simulink model "DMC_plant_velocity"  (R2022b)
settings: Solver=ode4  StartTime=0.0  StopTime=100  FixedStep=0.1  RelTol=1e-3  EnableMultiTasking=on
Description:
  | Real-Time Van der Pol Simulation
  | 
  | This demonstration shows a real-time version of the Simulink Van der Pol
  | simulation demo. This model does not need any external signals, so it does
  | not need any data acquisition hardware or driver. This makes the model ideal
  | for first experiments with Real-Time Windows Target, without need to
  | worry about proper I/O hardware configuration.
  | 
  | How to run this demo:
  | 
  |   1. Build the model using Tools -> Real-Time Workshop -> Build Model.
  |   2. Connect to the real-time code using Simulation -> Connect to target.
  |   3. Start the real-time execution using Simulation -> Start real-time code.
settings Model: SimulationMode=external  Creator=Houska  LastModifiedBy=artur
settings SolverCC: AlgebraicLoopSolver=TrustRegion
settings DataIOCC: LimitDataPoints=on  SaveFormat=Array  SignalLoggingSaveFormat=ModelDataLogs  SaveOutput=off  SaveTime=off  ReturnWorkspaceOutputs=off  SignalLoggingName=logsOut
settings OptimizationCC: ExpressionDepthLimit=2147483647  InitFltsAndDblsToZero=on
settings DebuggingCC: SaveWithParameterizedLinksMsg=none  UnderspecifiedInitializationDetection=Classic  MergeDetectMultiDrivingBlocksExec=none  SignalResolutionControl=TryResolveAllWithWarning  MultiTaskDSMMsg=warning  MultiTaskCondExecSysMsg=none  FcnCallInpInsideContextMsg=warning  UnconnectedInputMsg=warning  UnconnectedOutputMsg=warning  UnconnectedLineMsg=warning  AllowSymbolicDim=off  StateNameClashWarn=warning  PregeneratedLibrarySubsystemCodeDiagnostic=none  SFUnexpectedBacktrackingDiag=warning  SFNoUnconditionalDefaultTransitionDiag=warning  SFExecutionAtInitializationDiag=none  SFMachineParentedDataDiag=warning  ArithmeticOperatorsInVariantConditions=warning
settings HardwareCC: ProdBitPerPointer=32  ProdBitPerSizeT=32  ProdBitPerPtrDiffT=32  ProdLargestAtomicFloat=None  ProdWordSize=32  ProdHWDeviceType=32-bit Real-Time Windows Target  TargetHWDeviceType=32-bit Generic  ProdEqTarget=off
settings ModelReferenceCC: EnableRefExpFcnMdlSchedulingChecks=on  PropagateSignalLabelsOutOfModel=off
settings SFSimCC: SimUseLocalCustomCode=off  CustomCodeUndefinedFunction=UseInterfaceOnly
settings RTWCC: Description=servo (Visual C/C++)  SystemTargetFile=rtcon_servo_usb2.tlc  TemplateMakefile=servo_vc_usb2_x64.tmf  RTWUseLocalCustomCode=off  DLArmComputeVersion=19.05
settings CodeAppCC: StateflowObjectComments=on
settings STFCustomTargetCC: ModelReferenceCompliant=off  CombineOutputUpdateFcns=on  MatFileLogging=on  SystemTargetFile=rtcon_servo_usb2.tlc
settings GRTTargetCC: TargetLangStandard=C89/C90 (ANSI)  ModelReferenceCompliant=off  ParMdlRefBuildCompliant=off  CompOptLevelCompliant=off  ConcurrentExecutionCompliant=off  CPPClassGenCompliant=off  UseToolchainInfoCompliant=off  ExtMode=on  ExtModeMexFile=rtcon_ext_comm
settings ConfigComp: CovMetricSettings=dw  CovSaveCumulativeToWorkspaceVar=on  CovSaveSingleToWorkspaceVar=on  CovExternalEMLEnable=off  CovSFcnEnable=off

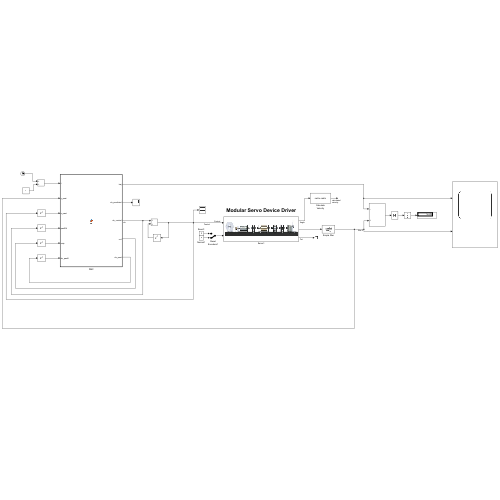
[thumbnail: Simulink's stored preview of the top-level diagram]
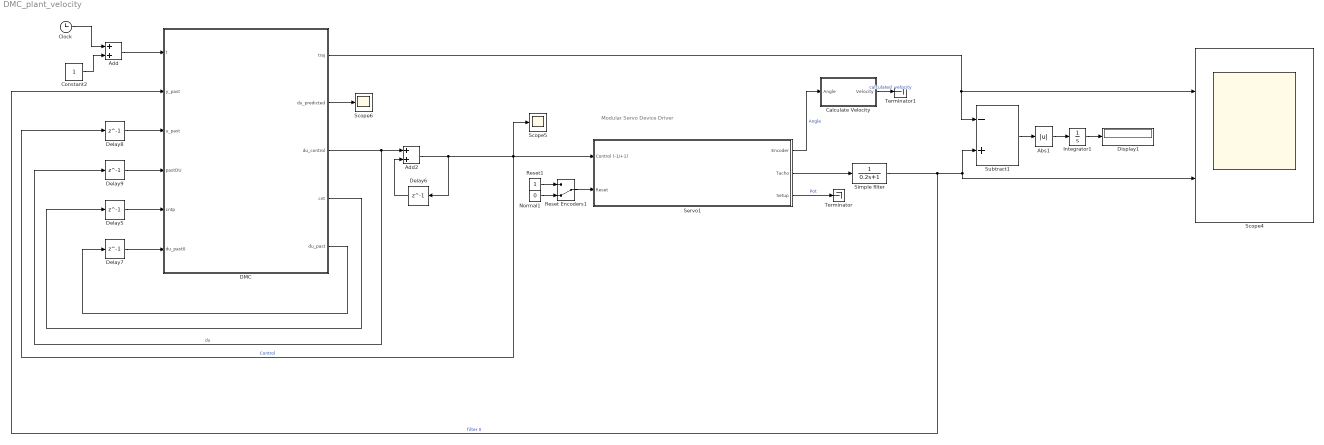
== system DMC_plant_velocity ==
  note: Modular Servo Device Driver
  Abs1 : Abs  SaturateOnIntegerOverflow=off
  Add : Sum
  Add2 : Sum
  Calculate Velocity : Subsystem
      mask Display: disp( 'rad-to-rad/s' )
  Clock : Clock
  Constant2 : Constant
  DMC : MATLAB Function  TreatAsAtomicUnit=on
  Delay5 : Delay  DelayLength=1  InitialCondition=1
  Delay6 : Delay  DelayLength=1  InitialCondition=0
  Delay7 : Delay  DelayLength=1  InitialCondition=zeros(1,150-1)
  Delay8 : Delay  DelayLength=1  InitialCondition=0
  Delay9 : Delay  DelayLength=1  InitialCondition=0
  Display1 : Display
  Integrator1 : Integrator
  Normal1 : Constant  Value=0
  Reset Encoders1 : ManualSwitch  CurrentSetting=0
  Reset1 : Constant
  Scope4 : Scope  NumInputPorts=2
  Scope5 : Scope
  Scope6 : Scope
  Servo1 : Subsystem
      mask Display: image(imread('Servo_inteco.JPG'))
  Simple filter : TransferFcn  Denominator=[0.2 1]
  Subtract1 : Sum  Inputs=-+
  Terminator : Terminator
  Terminator1 : Terminator
  wires:
  Delay8/1 -> DMC/3(u_past)
  Add/1 -> DMC/1(t)
  Integrator1/1 -> Display1/1
  Delay7/1 -> DMC/6(du_past0)
  Delay5/1 -> DMC/5(cntp)
  DMC/2(du_predicted) -> Scope6/1
  DMC/5(du_past) -> Delay7/1
  Servo1/2(Tacho) -> Simple filter/1
  DMC/3(du_control) -> Add2/1, Delay9/1  "du"
  Servo1/1(Encoder) -> Calculate Velocity/1(Angle)  "Angle"
  DMC/4(cnt) -> Delay5/1
  Delay6/1 -> Add2/2
  Delay9/1 -> DMC/4(pastDU)
  Abs1/1 -> Integrator1/1
  Subtract1/1 -> Abs1/1
  DMC/1(traj) -> Scope4/1, Subtract1/1
  Add2/1 -> Delay6/1, Servo1/1(Control (-1/+1)), Scope5/1, Delay8/1  "Control"
  Normal1/1 -> Reset Encoders1/2
  Reset1/1 -> Reset Encoders1/1
  Reset Encoders1/1 -> Servo1/2(Reset)
  Servo1/3(Setup) -> Terminator/1  "Pot"
  Constant2/1 -> Add/2
  Clock/1 -> Add/1
  Calculate Velocity/1(Velocity) -> Terminator1/1  "calculated  velocity"
  Simple filter/1 -> DMC/2(y_past), Scope4/2, Subtract1/2  "filter II"

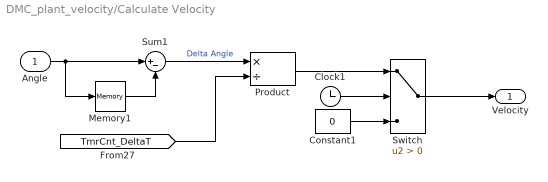
== system DMC_plant_velocity/Calculate Velocity ==
  Angle : Inport
  Clock1 : Clock
  Constant1 : Constant  Value=0
  Memory1 : Memory
  Product : Product  Inputs=*/  InputSameDT=on  SaturateOnIntegerOverflow=on  OutDataTypeStr=Inherit: Same as first input
  Sum1 : Sum  Inputs=|+-  InputSameDT=on  SaturateOnIntegerOverflow=on  OutDataTypeStr=Inherit: Same as first input
  Switch : Switch  Criteria=u2 > Threshold
  Velocity : Outport  VectorParamsAs1DForOutWhenUnconnected=off
  wires:
  Switch/1 -> Velocity/1
  Constant1/1 -> Switch/3
  Clock1/1 -> Switch/2
  Product/1 -> Switch/1
  Sum1/1 -> Product/1  "Delta Angle"
  Angle/1 -> Memory1/1, Sum1/1
  Memory1/1 -> Sum1/2
  [TmrCnt_DeltaT] -> Product/2

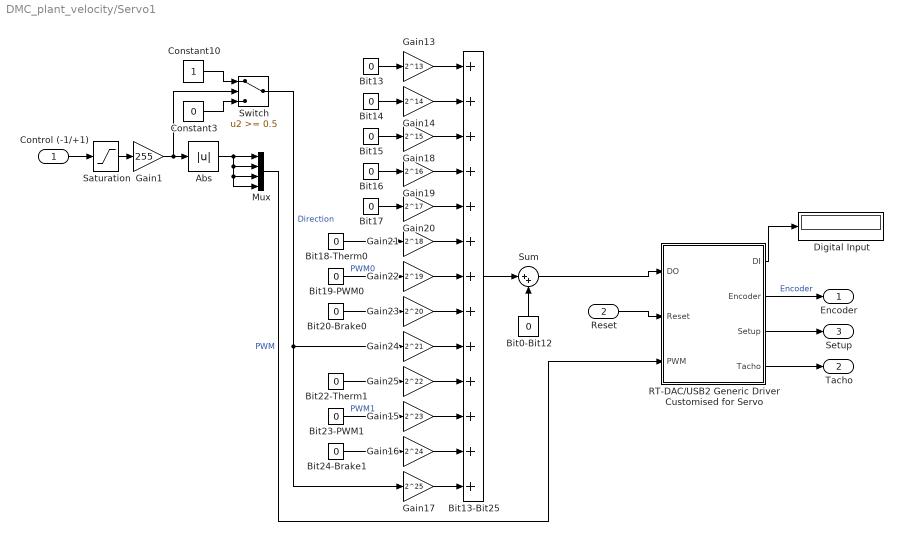
== system DMC_plant_velocity/Servo1 ==
  Control (-1/+1) : Inport
  Reset : Inport  Port=2
  Abs : Abs
  Bit0-Bit12 : Constant  Value=0
  Bit{13..17} (5 alike) : Constant  Value=0
  Bit13-Bit25 : Sum  Inputs=+++++++++++++  InputSameDT=on  SaturateOnIntegerOverflow=on  OutDataTypeStr=Inherit: Same as first input
  Bit18-Therm0 : Constant  Value=0
  Bit19-PWM0 : Constant  Value=0
  Bit20-Brake0 : Constant  Value=0
  Bit22-Therm1 : Constant  Value=0
  Bit23-PWM1 : Constant  Value=0
  Bit24-Brake1 : Constant  Value=0
  Constant10 : Constant
  Constant3 : Constant  Value=0
  Digital Input : Display
  Gain1 : Gain  Gain=255  SaturateOnIntegerOverflow=on  OutDataTypeStr=Inherit: Same as input  ParamDataTypeStr=Inherit: Same as input
  Gain13 : Gain  Gain=2^13  SaturateOnIntegerOverflow=on  OutDataTypeStr=Inherit: Same as input  ParamDataTypeStr=Inherit: Same as input
  Gain14 : Gain  Gain=2^14  SaturateOnIntegerOverflow=on  OutDataTypeStr=Inherit: Same as input  ParamDataTypeStr=Inherit: Same as input
  Gain15 : Gain  Gain=2^23  SaturateOnIntegerOverflow=on  OutDataTypeStr=Inherit: Same as input  ParamDataTypeStr=Inherit: Same as input
  Gain16 : Gain  Gain=2^24  SaturateOnIntegerOverflow=on  OutDataTypeStr=Inherit: Same as input  ParamDataTypeStr=Inherit: Same as input
  Gain17 : Gain  Gain=2^25  SaturateOnIntegerOverflow=on  OutDataTypeStr=Inherit: Same as input  ParamDataTypeStr=Inherit: Same as input
  Gain18 : Gain  Gain=2^15  SaturateOnIntegerOverflow=on  OutDataTypeStr=Inherit: Same as input  ParamDataTypeStr=Inherit: Same as input
  Gain19 : Gain  Gain=2^16  SaturateOnIntegerOverflow=on  OutDataTypeStr=Inherit: Same as input  ParamDataTypeStr=Inherit: Same as input
  Gain20 : Gain  Gain=2^17  SaturateOnIntegerOverflow=on  OutDataTypeStr=Inherit: Same as input  ParamDataTypeStr=Inherit: Same as input
  Gain21 : Gain  Gain=2^18  SaturateOnIntegerOverflow=on  OutDataTypeStr=Inherit: Same as input  ParamDataTypeStr=Inherit: Same as input
  Gain22 : Gain  Gain=2^19  SaturateOnIntegerOverflow=on  OutDataTypeStr=Inherit: Same as input  ParamDataTypeStr=Inherit: Same as input
  Gain23 : Gain  Gain=2^20  SaturateOnIntegerOverflow=on  OutDataTypeStr=Inherit: Same as input  ParamDataTypeStr=Inherit: Same as input
  Gain24 : Gain  Gain=2^21  SaturateOnIntegerOverflow=on  OutDataTypeStr=Inherit: Same as input  ParamDataTypeStr=Inherit: Same as input
  Gain25 : Gain  Gain=2^22  SaturateOnIntegerOverflow=on  OutDataTypeStr=Inherit: Same as input  ParamDataTypeStr=Inherit: Same as input
  Mux : Mux
  RT-DAC/USB2 Generic Driver Customised for Servo : Subsystem
      mask Display: disp('RT-DAC/USB2\n\nGeneric Driver\nVersion 2.1')
  Saturation : Saturate  UpperLimit=1  LowerLimit=-1
  Sum : Sum  Inputs=|++  InputSameDT=on  SaturateOnIntegerOverflow=on  OutDataTypeStr=Inherit: Same as first input
  Switch : Switch  Threshold=0.5  SaturateOnIntegerOverflow=off
  Encoder : Outport  VectorParamsAs1DForOutWhenUnconnected=off
  Tacho : Outport  Port=2  VectorParamsAs1DForOutWhenUnconnected=off
  Setup : Outport  Port=3  VectorParamsAs1DForOutWhenUnconnected=off
  wires:
  RT-DAC/USB2 Generic Driver Customised for Servo/4(Tacho) -> Tacho/1
  RT-DAC/USB2 Generic Driver Customised for Servo/3(Setup) -> Setup/1
  RT-DAC/USB2 Generic Driver Customised for Servo/2(Encoder) -> Encoder/1  "Encoder"
  Mux/1 -> RT-DAC/USB2 Generic Driver Customised for Servo/3(PWM)  "PWM"
  Switch/1 -> Gain17/1, Gain24/1  "Direction"
  Abs/1 -> Mux/4, Mux/3, Mux/2, Mux/1
  Constant3/1 -> Switch/3
  Constant10/1 -> Switch/1
  Gain1/1 -> Switch/2, Abs/1
  Saturation/1 -> Gain1/1
  Control (-1/+1)/1 -> Saturation/1
  Reset/1 -> RT-DAC/USB2 Generic Driver Customised for Servo/2(Reset)
  Bit24-Brake1/1 -> Gain16/1
  Bit23-PWM1/1 -> Gain15/1  "PWM1"
  Bit22-Therm1/1 -> Gain25/1
  Bit13-Bit25/1 -> Sum/1
  Sum/1 -> RT-DAC/USB2 Generic Driver Customised for Servo/1(DO)
  Gain17/1 -> Bit13-Bit25/13
  Gain16/1 -> Bit13-Bit25/12
  Gain15/1 -> Bit13-Bit25/11
  Gain25/1 -> Bit13-Bit25/10
  Gain24/1 -> Bit13-Bit25/9
  Gain23/1 -> Bit13-Bit25/8
  Gain22/1 -> Bit13-Bit25/7
  Gain21/1 -> Bit13-Bit25/6
  Gain20/1 -> Bit13-Bit25/5
  Gain19/1 -> Bit13-Bit25/4
  Gain18/1 -> Bit13-Bit25/3
  Gain14/1 -> Bit13-Bit25/2
  Gain13/1 -> Bit13-Bit25/1
  Bit0-Bit12/1 -> Sum/2
  RT-DAC/USB2 Generic Driver Customised for Servo/1(DI) -> Digital Input/1
  Bit20-Brake0/1 -> Gain23/1
  Bit19-PWM0/1 -> Gain22/1  "PWM0"
  Bit18-Therm0/1 -> Gain21/1
  Bit17/1 -> Gain20/1
  Bit16/1 -> Gain19/1
  Bit15/1 -> Gain18/1
  Bit14/1 -> Gain14/1
  Bit13/1 -> Gain13/1

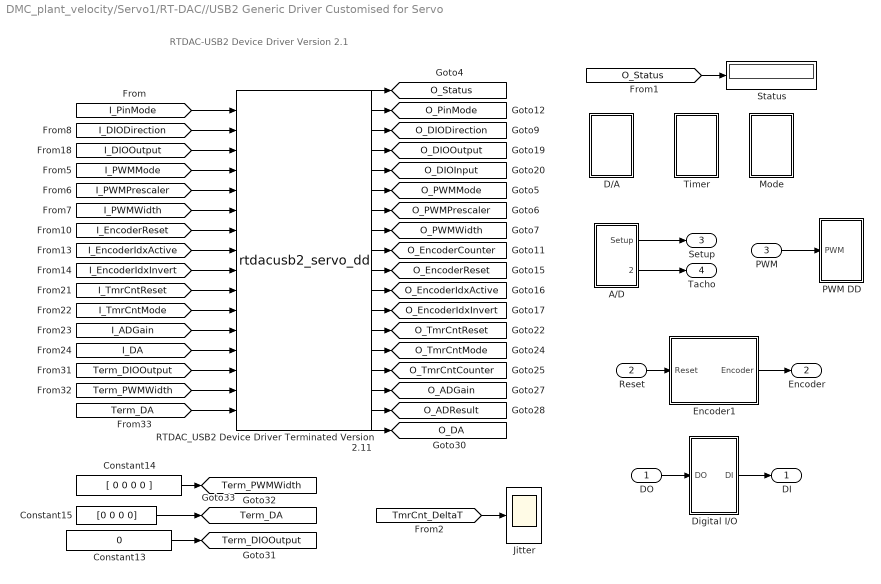
== system DMC_plant_velocity/Servo1/RT-DAC//USB2 Generic Driver Customised for Servo ==
  note: RTDAC-USB2 Device Driver
      | Version 2.1
  DO : Inport
  Reset : Inport  Port=2
  PWM : Inport  Port=3
  A/D : Subsystem
  Constant13 : Constant  Value=0
  Constant14 : Constant  Value=[ 0 0 0 0 ]
  Constant15 : Constant  Value=[0 0 0 0]
  D/A : Subsystem
  Digital I/O : Subsystem
  Encoder1 : Subsystem
  Jitter : Scope
  Mode : Subsystem
  PWM DD : Subsystem
  RTDAC_USB2 Device Driver Terminated Version 2.11 : S-Function  FunctionName=rtdacusb2_servo_dd  Parameters=0.1  SFunctionDeploymentMode=off  EnableBusSupport=off
  Status : Display
  Timer : Subsystem
  DI : Outport  VectorParamsAs1DForOutWhenUnconnected=off
  Encoder : Outport  Port=2  VectorParamsAs1DForOutWhenUnconnected=off
  Setup : Outport  Port=3  VectorParamsAs1DForOutWhenUnconnected=off
  Tacho : Outport  Port=4  VectorParamsAs1DForOutWhenUnconnected=off
  tag scope: O_ADGain=global, O_ADResult=global, O_DA=global, O_DIODirection=global, O_DIOInput=global, O_DIOOutput=global, O_EncoderCounter=global, O_EncoderIdxActive=global, O_EncoderIdxInvert=global, O_EncoderReset=global, O_PWMMode=global, O_PWMPrescaler=global, O_PWMWidth=global, O_PinMode=global, O_Status=global, O_TmrCntCounter=global, O_TmrCntMode=global, O_TmrCntReset=global, Term_DA=global, Term_DIOOutput=global, Term_PWMWidth=global
  wires:
  [TmrCnt_DeltaT] -> Jitter/1
  Constant14/1 -> [Term_PWMWidth]
  [Term_DA] -> RTDAC_USB2 Device Driver Terminated Version 2.11/16
  [Term_PWMWidth] -> RTDAC_USB2 Device Driver Terminated Version 2.11/15
  [Term_DIOOutput] -> RTDAC_USB2 Device Driver Terminated Version 2.11/14
  Constant13/1 -> [Term_DIOOutput]
  Constant15/1 -> [Term_DA]
  A/D/2(Tacho) -> Tacho/1
  A/D/1(Setup) -> Setup/1
  Reset/1 -> Encoder1/1(Reset)
  Digital I/O/1(DI) -> DI/1
  DO/1 -> Digital I/O/1(DO)
  Encoder1/1(Encoder) -> Encoder/1
  RTDAC_USB2 Device Driver Terminated Version 2.11/5 -> [O_DIOInput]
  RTDAC_USB2 Device Driver Terminated Version 2.11/4 -> [O_DIOOutput]
  [I_DIOOutput] -> RTDAC_USB2 Device Driver Terminated Version 2.11/3
  RTDAC_USB2 Device Driver Terminated Version 2.11/12 -> [O_EncoderIdxInvert]
  RTDAC_USB2 Device Driver Terminated Version 2.11/11 -> [O_EncoderIdxActive]
  RTDAC_USB2 Device Driver Terminated Version 2.11/10 -> [O_EncoderReset]
  [I_EncoderIdxInvert] -> RTDAC_USB2 Device Driver Terminated Version 2.11/9
  [I_EncoderIdxActive] -> RTDAC_USB2 Device Driver Terminated Version 2.11/8
  RTDAC_USB2 Device Driver Terminated Version 2.11/2 -> [O_PinMode]
  RTDAC_USB2 Device Driver Terminated Version 2.11/3 -> [O_DIODirection]
  RTDAC_USB2 Device Driver Terminated Version 2.11/9 -> [O_EncoderCounter]
  [I_EncoderReset] -> RTDAC_USB2 Device Driver Terminated Version 2.11/7
  [I_DIODirection] -> RTDAC_USB2 Device Driver Terminated Version 2.11/2
  [I_PWMWidth] -> RTDAC_USB2 Device Driver Terminated Version 2.11/6
  [I_PWMPrescaler] -> RTDAC_USB2 Device Driver Terminated Version 2.11/5
  [I_PWMMode] -> RTDAC_USB2 Device Driver Terminated Version 2.11/4
  RTDAC_USB2 Device Driver Terminated Version 2.11/8 -> [O_PWMWidth]
  RTDAC_USB2 Device Driver Terminated Version 2.11/7 -> [O_PWMPrescaler]
  RTDAC_USB2 Device Driver Terminated Version 2.11/6 -> [O_PWMMode]
  [O_Status] -> Status/1
  RTDAC_USB2 Device Driver Terminated Version 2.11/1 -> [O_Status]
  PWM/1 -> PWM DD/1(PWM)
  [I_PinMode] -> RTDAC_USB2 Device Driver Terminated Version 2.11/1
  [I_TmrCntReset] -> RTDAC_USB2 Device Driver Terminated Version 2.11/10
  [I_ADGain] -> RTDAC_USB2 Device Driver Terminated Version 2.11/12
  [I_TmrCntMode] -> RTDAC_USB2 Device Driver Terminated Version 2.11/11
  [I_DA] -> RTDAC_USB2 Device Driver Terminated Version 2.11/13
  RTDAC_USB2 Device Driver Terminated Version 2.11/13 -> [O_TmrCntReset]
  RTDAC_USB2 Device Driver Terminated Version 2.11/14 -> [O_TmrCntMode]
  RTDAC_USB2 Device Driver Terminated Version 2.11/15 -> [O_TmrCntCounter]
  RTDAC_USB2 Device Driver Terminated Version 2.11/16 -> [O_ADGain]
  RTDAC_USB2 Device Driver Terminated Version 2.11/17 -> [O_ADResult]
  RTDAC_USB2 Device Driver Terminated Version 2.11/18 -> [O_DA]

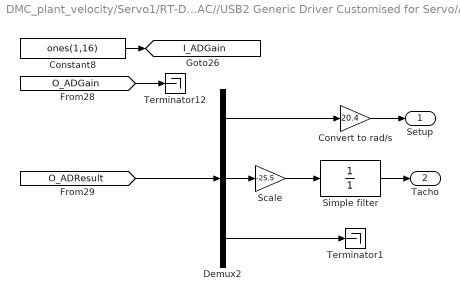
== system DMC_plant_velocity/Servo1/RT-DAC//USB2 Generic Driver Customised for Servo/A//D ==
  Constant8 : Constant  Value=ones(1,16)
  Convert to rad/s : Gain  Gain=20.4  OutDataTypeStr=Inherit: Same as input  ParamDataTypeStr=Inherit: Same as input
  Demux2 : Demux  Outputs=[1 1 14]
      settings: DisplayOption=none
  Scale : Gain  Gain=-25.5  OutDataTypeStr=Inherit: Same as input  ParamDataTypeStr=Inherit: Same as input
  Simple filter : TransferFcn  Denominator=[0.0 1]
  Terminator1 : Terminator
  Terminator12 : Terminator
  Setup : Outport  InitialOutput=0  VectorParamsAs1DForOutWhenUnconnected=off
  Tacho : Outport  Port=2  InitialOutput=0  VectorParamsAs1DForOutWhenUnconnected=off
  tag scope: I_ADGain=global
  wires:
  Scale/1 -> Simple filter/1
  Demux2/3 -> Terminator1/1
  Simple filter/1 -> Tacho/1
  Convert to rad/s/1 -> Setup/1
  Demux2/1 -> Convert to rad/s/1
  Demux2/2 -> Scale/1
  Constant8/1 -> [I_ADGain]
  [O_ADGain] -> Terminator12/1
  [O_ADResult] -> Demux2/1

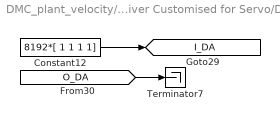
== system DMC_plant_velocity/Servo1/RT-DAC//USB2 Generic Driver Customised for Servo/D//A ==
  Constant12 : Constant  Value=8192*[ 1 1 1 1]
  Terminator7 : Terminator
  tag scope: I_DA=global
  wires:
  [O_DA] -> Terminator7/1
  Constant12/1 -> [I_DA]

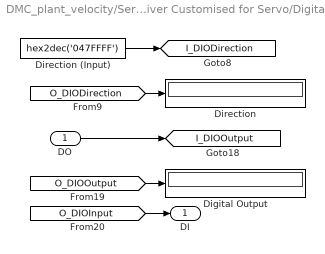
== system DMC_plant_velocity/Servo1/RT-DAC//USB2 Generic Driver Customised for Servo/Digital I//O ==
  DO : Inport
  Digital Output : Display
  Direction : Display
  Direction (Input) : Constant  Value=hex2dec('047FFFF')
  DI : Outport  VectorParamsAs1DForOutWhenUnconnected=off
  tag scope: I_DIODirection=global, I_DIOOutput=global
  wires:
  [O_DIOInput] -> DI/1
  [O_DIOOutput] -> Digital Output/1
  DO/1 -> [I_DIOOutput]
  [O_DIODirection] -> Direction/1
  Direction (Input)/1 -> [I_DIODirection]

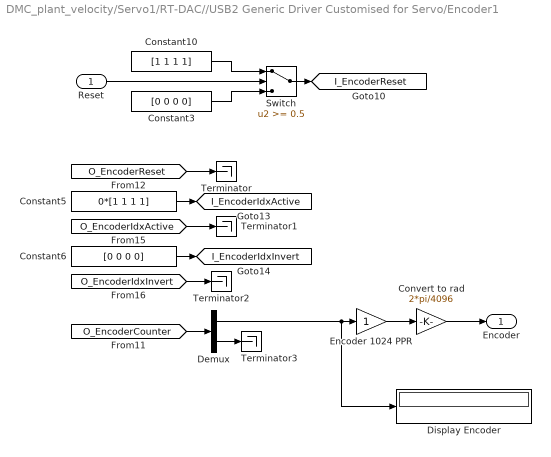
== system DMC_plant_velocity/Servo1/RT-DAC//USB2 Generic Driver Customised for Servo/Encoder1 ==
  Reset : Inport
  Constant10 : Constant  Value=[1 1 1 1]
  Constant3 : Constant  Value=[0 0 0 0]
  Constant5 : Constant  Value=0*[1 1 1 1]
  Constant6 : Constant  Value=[0 0 0 0]
  Convert to rad : Gain  Gain=2*pi/4096  SaturateOnIntegerOverflow=on  OutDataTypeStr=Inherit: Same as input  ParamDataTypeStr=Inherit: Same as input
  Demux : Demux  Outputs=[1 3]
  Display Encoder : Display
  Encoder 1024 PPR : Gain  SaturateOnIntegerOverflow=on  OutDataTypeStr=Inherit: Same as input  ParamDataTypeStr=Inherit: Same as input
  Switch : Switch  Threshold=0.5  SaturateOnIntegerOverflow=off
  Terminator{,1..3} (4 alike) : Terminator
  Encoder : Outport  VectorParamsAs1DForOutWhenUnconnected=off
  tag scope: I_EncoderIdxActive=global, I_EncoderIdxInvert=global, I_EncoderReset=global
  wires:
  Convert to rad/1 -> Encoder/1
  Demux/1 -> Encoder 1024 PPR/1, Display Encoder/1
  Encoder 1024 PPR/1 -> Convert to rad/1
  Reset/1 -> Switch/2
  Constant3/1 -> Switch/3
  Constant10/1 -> Switch/1
  Switch/1 -> [I_EncoderReset]
  Demux/2 -> Terminator3/1
  [O_EncoderIdxInvert] -> Terminator2/1
  [O_EncoderIdxActive] -> Terminator1/1
  Constant6/1 -> [I_EncoderIdxInvert]
  Constant5/1 -> [I_EncoderIdxActive]
  [O_EncoderReset] -> Terminator/1
  [O_EncoderCounter] -> Demux/1

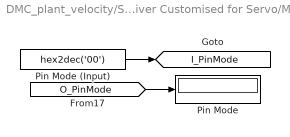
== system DMC_plant_velocity/Servo1/RT-DAC//USB2 Generic Driver Customised for Servo/Mode ==
  Pin Mode : Display
  Pin Mode (Input) : Constant  Value=hex2dec('00')
  tag scope: I_PinMode=global
  wires:
  Pin Mode (Input)/1 -> [I_PinMode]
  [O_PinMode] -> Pin Mode/1

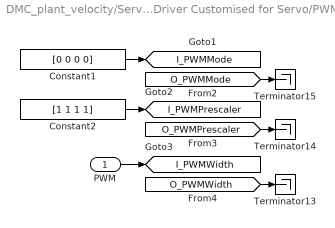
== system DMC_plant_velocity/Servo1/RT-DAC//USB2 Generic Driver Customised for Servo/PWM DD ==
  PWM : Inport
  Constant1 : Constant  Value=[0 0 0 0]
  Constant2 : Constant  Value=[1 1 1 1]
  Terminator13 : Terminator
  Terminator14 : Terminator
  Terminator15 : Terminator
  tag scope: I_PWMMode=global, I_PWMPrescaler=global, I_PWMWidth=global
  wires:
  PWM/1 -> [I_PWMWidth]
  [O_PWMWidth] -> Terminator13/1
  [O_PWMPrescaler] -> Terminator14/1
  [O_PWMMode] -> Terminator15/1
  Constant2/1 -> [I_PWMPrescaler]
  Constant1/1 -> [I_PWMMode]

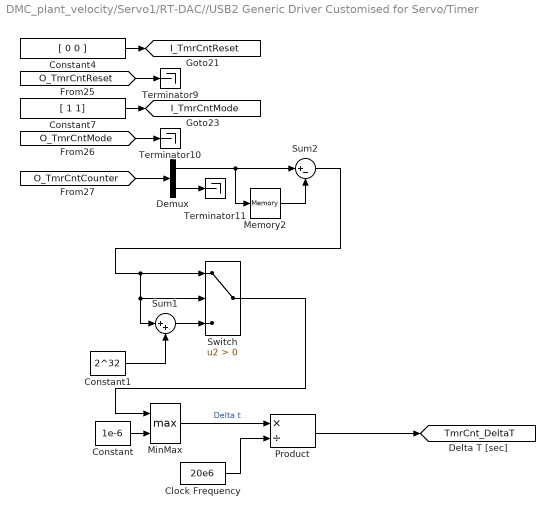
== system DMC_plant_velocity/Servo1/RT-DAC//USB2 Generic Driver Customised for Servo/Timer ==
  Clock Frequency : Constant  Value=20e6
  Constant : Constant  Value=1e-6
  Constant1 : Constant  Value=2^32
  Constant4 : Constant  Value=[ 0 0 ]
  Constant7 : Constant  Value=[ 1 1]
  Demux : Demux  Outputs=2
      settings: DisplayOption=none
  Memory2 : Memory
  MinMax : MinMax  Function=max  Inputs=2  InputSameDT=on  SaturateOnIntegerOverflow=on
  Product : Product  Inputs=*/  SaturateOnIntegerOverflow=on  OutDataTypeStr=Inherit: Same as first input
  Sum1 : Sum  Inputs=|++  InputSameDT=on  SaturateOnIntegerOverflow=on  OutDataTypeStr=Inherit: Same as first input
  Sum2 : Sum  Inputs=|+-  InputSameDT=on  SaturateOnIntegerOverflow=on  OutDataTypeStr=Inherit: Same as first input
  Switch : Switch  Criteria=u2 > Threshold
  Terminator10 : Terminator
  Terminator11 : Terminator
  Terminator9 : Terminator
  tag scope: I_TmrCntMode=global, I_TmrCntReset=global, TmrCnt_DeltaT=global
  wires:
  Demux/2 -> Terminator11/1
  Demux/1 -> Sum2/1, Memory2/1
  Switch/1 -> MinMax/1
  Constant1/1 -> Sum1/2
  Sum1/1 -> Switch/3
  Sum2/1 -> Sum1/1, Switch/2, Switch/1
  Clock Frequency/1 -> Product/2
  MinMax/1 -> Product/1  "Delta t"
  Product/1 -> [TmrCnt_DeltaT]
  [O_TmrCntCounter] -> Demux/1
  Memory2/1 -> Sum2/2
  Constant/1 -> MinMax/2
  Constant4/1 -> [I_TmrCntReset]
  [O_TmrCntReset] -> Terminator9/1
  Constant7/1 -> [I_TmrCntMode]
  [O_TmrCntMode] -> Terminator10/1

== matlab function DMC_plant_velocity/DMC ==
  data: traj output; du_predicted output; t input; y_past input; u_past input; pastDU input; du_control output; cntp input; cnt output; du_past0 input; du_past output
function [traj,du_predicted, du_control,cnt,du_past] = fcn(t,y_past,u_past,pastDU,cntp,du_past0)

cnt = cntp;
    
%Parametry
    ny = 60; %HORYZONT PREDYKCJI
    nu = 20; %HORYZONT STEROWANIA
    lambda = 10;
    D = 150;
    gi = [0	13.8890714485793	26.5164102416302	37.9966366617195	48.4339584772272	57.9231168521736	66.5502463262337	74.3936566711070	81.5245437202744	88.0076356244511	93.9017803988952	99.2604800958292	104.132376450738	108.561692410831	112.588633553487	116.249753038417	119.578283406283	122.604438235539	125.355686395700	127.857001386462	130.131088025978	132.198588545954	134.078269964341	135.787194436423	137.340874130607	138.753412034740	140.037629971091	141.205184981981	142.266675142546	143.231735761073	144.109126840174	144.906812592661	145.632033733925	146.291373207016	146.890815937020	147.435803157138	147.931281799595	148.381749399691	148.791294920627	149.163635869636	149.502152042375	149.809916201839	150.089721970301	150.344109187453	150.575386964913	150.785654646384	150.976820863722	151.150620861876	151.308632249969	151.452289321502	151.582896073651	151.701638043850	151.809593071097	151.907741079659	151.996972973999	152.078098725648	152.151854725443	152.218910467857	152.279874628106	152.335300587180	152.385691454974	152.431504637092	152.473155986783	152.511023579709	152.545451145794	152.576751189313	152.605207825541	152.631079359709	152.654600631686	152.675985147648	152.695427018113	152.713102719908	152.729172698077	152.743782822266	152.757065710804	152.769141934498	152.780121111075	152.790102900198	152.799177908090	152.807428509985	152.814929597855	152.821749260220	152.827949400198	152.833586297406	152.838711118820	152.843370383227	152.847606383482	152.851457570406	152.854958901810	152.858142159815	152.861036239340	152.863667410386	152.866059556495	152.868234391542	152.870211656837	152.872009300320	152.873643639474	152.875129509446	152.876480397704	152.877708566467	152.878825164011	152.879840325863	152.880763266801	152.881602364501	152.882365235581	152.883058804738	152.883689367607	152.884262647901	152.884783849374	152.885257703051	152.885688510175	152.886080181247	152.886436271526	152.886760013297	152.887054345214	152.887321938973	152.887565223563	152.887786407315	152.887987497949	152.888170320794	152.888336535361	152.888487650406	152.888625037623	152.888749944096	152.888863503621	152.888966746995	152.889060611373	152.889145948778	152.889223533829	152.889294070778	152.889358199899	152.889416503303	152.889469510219	152.889517701797	152.889561515482	152.889601348975	152.889637563852	152.889670488841	152.889700422807	152.889727637465	152.889752379846	152.889774874542	152.889795325739	152.889813919077	152.889830823330	152.889846191941	152.889860164412	152.889872867574	152.889884416736	152.889894916731	152.889904462869	152.889913141801	152.889921032309	152.889928206015	152.889934728036	152.889940657573	152.889946048451	152.889950949601	152.889955405514	152.889959456636	152.889963139739	152.889966488256	152.889969532582	152.889972300351	152.889974816685	152.889977104427	152.889979184343	152.889981075311	152.889982794497	152.889984357506	152.889985778526	152.889987070455	152.889988245021	152.889989312885	152.889990283741	152.889991166400	152.889991968876	152.889992698452	152.889993361750	152.889993964792	152.889994513052	152.889995011506	152.889995464679	152.889995876683	152.889996251260	152.889996591809	152.889996901421	152.889997182907	152.889997438822	152.889997671488	152.889997883019	152.889998075333	152.889998250176	152.889998409136	152.889998553656	152.889998685047	152.889998804502	152.889998913105	152.889999011843	152.889999101610	152.889999183223	152.889999257422	152.889999324881	152.889999386211	152.889999441970	152.889999492663	152.889999538751	152.889999580653	152.889999618748	152.889999653382	152.889999684870	152.889999713498	152.889999739524	152.889999763187	152.889999784700	152.889999804259	152.889999822040	152.889999838207	152.889999852905	152.889999866267	152.889999878416	152.889999889461	152.889999899503	152.889999908632	152.889999916933	152.889999924479	152.889999931339	152.889999937577	152.889999943247	152.889999948403	152.889999953090	152.889999957352	152.889999961226	152.889999964748	152.889999967951	152.889999970862	152.889999973509	152.889999975916	152.889999978104	152.889999980093	152.889999981901	152.889999983545	152.889999985040	152.889999986399	152.889999987635	152.889999988758	152.889999989779	152.889999990708	152.889999991552	152.889999992319	152.889999993017	152.889999993651	152.889999994228	152.889999994752	152.889999995229	152.889999995662	152.889999996056	152.889999996415	152.889999996740	152.889999997036	152.889999997306	152.889999997550	152.889999997773	152.889999997975	152.889999998159	152.889999998326	152.889999998478	152.889999998617	152.889999998742	152.889999998857	152.889999998960	152.889999999055	152.889999999141	152.889999999219	152.889999999290	152.889999999354	152.889999999413	152.889999999466	152.889999999515	152.889999999559	152.889999999599	152.889999999635	152.889999999668	152.889999999699	152.889999999726	152.889999999751	152.889999999773	152.889999999794	152.889999999813	152.889999999830	152.889999999845	152.889999999859	152.889999999872	152.889999999884	152.889999999894	152.889999999904	152.889999999913	152.889999999920	152.889999999928	152.889999999934	152.889999999940	152.889999999946	152.889999999951	152.889999999955	152.889999999959	152.889999999963	152.889999999966	152.889999999969	152.889999999972	152.889999999975	152.889999999977	152.889999999979	152.889999999981	152.889999999983	152.889999999984	152.889999999986	152.889999999987	152.889999999988	152.889999999989	152.889999999990	152.889999999991	152.889999999992	152.889999999993	152.889999999993	152.889999999994	152.889999999994	152.889999999995	152.889999999995	152.889999999996	152.889999999996	152.889999999996	152.889999999997	152.889999999997	152.889999999997	152.889999999997	152.889999999998	152.889999999998	152.889999999998	152.889999999998	152.889999999998	152.889999999999	152.889999999999	152.889999999999	152.889999999999	152.889999999999	152.889999999999	152.889999999999	152.889999999999	152.889999999999	152.889999999999	152.889999999999	152.889999999999	152.889999999999	152.889999999999	152.889999999999	152.890000000000	152.890000000000	152.890000000000	152.890000000000	152.890000000000	152.890000000000	152.890000000000	152.890000000000	152.890000000000	152.890000000000	152.890000000000	152.890000000000	152.890000000000	152.890000000000	152.890000000000	152.890000000000	152.890000000000	152.890000000000	152.890000000000	152.890000000000	152.890000000000	152.890000000000	152.890000000000	152.890000000000	152.890000000000	152.890000000000	152.890000000000	152.890000000000	152.890000000000	152.890000000000	152.890000000000	152.890000000000	152.890000000000	152.890000000000	152.890000000000	152.890000000000	152.890000000000	152.890000000000	152.890000000000	152.890000000000	152.890000000000	152.890000000000	152.890000000000	152.890000000000	152.890000000000	152.890000000000	152.890000000000	152.890000000000	152.890000000000	152.890000000000	152.890000000000	152.890000000000	152.890000000000	152.890000000000	152.890000000000	152.890000000000	152.890000000000	152.890000000000	152.890000000000	152.890000000000	152.890000000000	152.890000000000	152.890000000000	152.890000000000	152.890000000000	152.890000000000	152.890000000000	152.890000000000	152.890000000000	152.890000000000	152.890000000000	152.890000000000	152.890000000000	152.890000000000	152.890000000000	152.890000000000	152.890000000000	152.890000000000	152.890000000000	152.890000000000	152.890000000000	152.890000000000	152.890000000000	152.890000000000	152.890000000000	152.890000000000	152.890000000000	152.890000000000	152.890000000000	152.890000000000	152.890000000000	152.890000000000	152.890000000000	152.890000000000	152.890000000000	152.890000000000	152.890000000000	152.890000000000	152.890000000000	152.890000000000	152.890000000000	152.890000000000	152.890000000000	152.890000000000	152.890000000000	152.890000000000	152.890000000000	152.890000000000	152.890000000000	152.890000000000	152.890000000000	152.890000000000	152.890000000000	152.890000000000	152.890000000000	152.890000000000	152.890000000000	152.890000000000	152.890000000000	152.890000000000	152.890000000000	152.890000000000	152.890000000000	152.890000000000	152.890000000000	152.890000000000	152.890000000000	152.890000000000	152.890000000000	152.890000000000	152.890000000000	152.890000000000	152.890000000000	152.890000000000	152.890000000000	152.890000000000	152.890000000000	152.890000000000	152.890000000000	152.890000000000	152.890000000000	152.890000000000	152.890000000000	152.890000000000	152.890000000000	152.890000000000];
    ograniczenie_wyjscia = false;
    
%Wektor przeszłych du
for i = 1:D-2
    du_past0(D-i) = du_past0(D-1-i);
end

du_past0(1) = pastDU;
du_past = du_past0;


% %Ustawienie ograniczeń dla optymalizatora 
    du_max = 1;
    du_min = -1;
    u_max = 1;
    u_min = -1;
    y_max = 42;
    y_min = -42;

%Trajektoria referencyjna, stała
Ts = 0.1; sim_time = 100; ref = 100;

traj_ub = ref*ones(1/Ts*sim_time/2,1);

traj_lb = -ref*ones(1/Ts*sim_time/2,1);

trajektoria = [traj_ub;traj_lb;traj_lb;-ref*ones(ny,1)];

ref = trajektoria(fix(t/Ts):ny+fix(t/Ts)-1, 1);

traj = ref(1);

    
%Wyznaczenie macierzy predykcji
    
    [H,P] = dmc_predmat(ny,nu,D,gi);
    Q = ones(ny,1);
    
%Prawo sterowania dla algorytmu z ograniczeniami
    S = H'*H + eye(nu)*lambda;
    S = (S + S')/2;
    f = H'*Q * y_past + H'*P * du_past - H' * ref;

%OGRANICZENIA
    if ograniczenie_wyjscia == true
        %OGRANICZENIA Z Y
        [C,dd,du,ddu,dy] = mpc_ograniczenia(du_max,du_min,u_max,u_min,y_max,y_min,nu,H,P,Q,D-1,1);
        dt = dd + du * u_past + ddu * du_past + dy*y_past;
    else
        %OGRANICZENIA BEZ Y
        [C, dd,du] = mpc_ograniczenia_bez_y(du_max,du_min,u_max,u_min,nu);
        dt = dd + du * u_past;
    end

    opts = optimoptions('quadprog','Algorithm','active-set');

    x0 = 1*eye(nu,1);

    du_predicted = quadprog(S,f,C,dt,[],[],[],[],x0,opts);

    du_control = du_predicted(1);

%Prawo sterowania dla algorytmu bez ograniczeń
% Pr = ( inv(H'*H+lambda*eye(nu)) ) * H';
% Nk = Pr*Q;
% Dk = Pr*P;
% 
% du_predicted = Pr * ref - Dk * du_past - Nk*y_past;
% du_control = du_predicted(1);

%Alternatywne prawo sterowania
% G = H;
% w = ref;
% f = Q *y_past + P * du_past;
% 
% du_predicted = inv(G' * G + lambda*eye(nu) ) * G' * (w - f);
% du_control = du_predicted(1);
